simulink model "SCAP_Obs"  (R2019b)
settings: Solver=FixedStepAuto  StartTime=0.0  StopTime=60  FixedStep=1e-3  RelTol=1e-3
libraries: simulink x1
settings Model: EnablePacing=on  PacingRate=5  Creator=lenovo  LastModifiedBy=19398

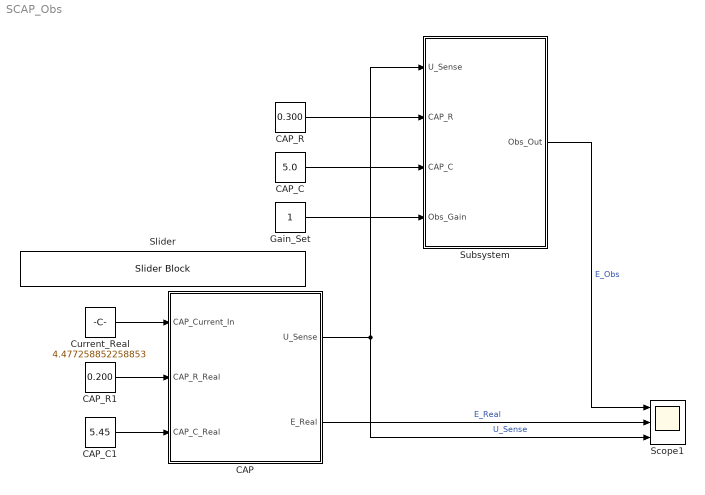
== system SCAP_Obs ==
  CAP : Subsystem
  CAP_C : Constant  Value=5.0
  CAP_C1 : Constant  Value=5.45
  CAP_R : Constant  Value=0.300
  CAP_R1 : Constant  Value=0.200
  Current_Real : Constant  Value=4.477258852258853
  Gain_Set : Constant
  Scope1 : Scope  NumInputPorts=3
  Slider : SliderBlock  ScaleMin=-20  ScaleMax=20
  Subsystem : Subsystem
  wires:
  CAP/1(U_Sense) -> Subsystem/1(U_Sense), Scope1/3  "U_Sense"
  CAP_R/1 -> Subsystem/2(CAP_R)
  CAP_C/1 -> Subsystem/3(CAP_C)
  Gain_Set/1 -> Subsystem/4(Obs_Gain)
  Current_Real/1 -> CAP/1(CAP_Current_In)
  CAP_R1/1 -> CAP/2(CAP_R_Real)
  CAP_C1/1 -> CAP/3(CAP_C_Real)
  Subsystem/1(Obs_Out) -> Scope1/1  "E_Obs"
  CAP/2(E_Real) -> Scope1/2  "E_Real"

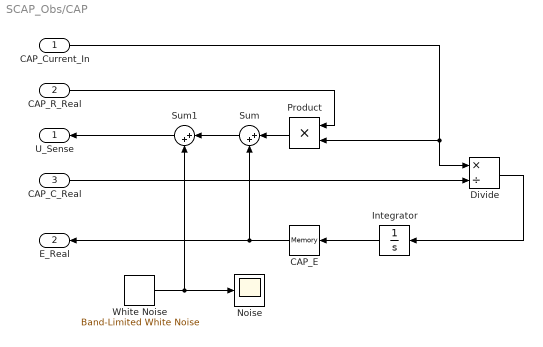
== system SCAP_Obs/CAP ==
  CAP_Current_In : Inport
  CAP_R_Real : Inport  Port=2
  CAP_C_Real : Inport  Port=3
  CAP_E : Memory
  Divide : Product  Inputs=*/
  Integrator : Integrator  InitialCondition=25
  Noise : Scope
  Product : Product
  Sum : Sum  Inputs=|++
  Sum1 : Sum  Inputs=|++
  White Noise : simulink/Sources/Band-Limited White Noise  Cov=0.002  Ts=1/10  seed=[23341]
  U_Sense : Outport
  E_Real : Outport  Port=2
  wires:
  CAP_C_Real/1 -> Divide/2
  Integrator/1 -> CAP_E/1
  CAP_E/1 -> Sum/2, E_Real/1
  CAP_Current_In/1 -> Product/2, Divide/1
  CAP_R_Real/1 -> Product/1
  Divide/1 -> Integrator/1
  Product/1 -> Sum/1
  Sum1/1 -> U_Sense/1
  White Noise/1 -> Noise/1, Sum1/2
  Sum/1 -> Sum1/1

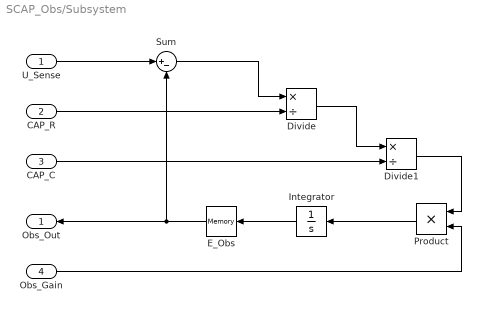
== system SCAP_Obs/Subsystem ==
  U_Sense : Inport
  CAP_R : Inport  Port=2
  CAP_C : Inport  Port=3
  Obs_Gain : Inport  Port=4
  Divide : Product  Inputs=*/
  Divide1 : Product  Inputs=*/
  E_Obs : Memory
  Integrator : Integrator
  Product : Product
  Sum : Sum  Inputs=|+-
  Obs_Out : Outport
  wires:
  E_Obs/1 -> Sum/2, Obs_Out/1
  Integrator/1 -> E_Obs/1
  Divide/1 -> Divide1/1
  Sum/1 -> Divide/1
  Divide1/1 -> Product/1
  CAP_R/1 -> Divide/2
  CAP_C/1 -> Divide1/2
  U_Sense/1 -> Sum/1
  Obs_Gain/1 -> Product/2
  Product/1 -> Integrator/1
